simulink model "LoFT_Example3"  (R2024b)
settings: Solver=ode4  StartTime=0.0  StopTime=300  FixedStep=simu.dt  RelTol=1e-3
undefined symbols (not defined in the file): body, circtime, Communication, D1, Delta, irkb, line, LoFT, p0, Pn, s, simu, trip_time, Turbwind, waves, wind
libraries: simulink x350, spsThreePhaseVIMeasurementLib x41, spsThreePhasePISectionLineLib x34, spsThreePhaseParallelRLCLoadLib x21, spsThreePhaseTransformerTwoWindingsLib x14, spsLoadFlowBusLib x10, spsThreePhaseDynamicLoadLib x9, spsSynchronousMachinepuStandardLib x7, spsExcitationSystemLib x7, spsSteamTurbineandGovernorLib x7, spsGenericPowerSystemStabilizerLib x7, spsMultiBandPowerSystemStabilizerLib x7
(part 48 of 49)

== system LoFT_Example3/Onshore grid/Onshore Grid/Subsystem/SG9/Regulators9/Turbine  & Excitation Regulators Mac2/Stabilisateur ==
  Pm : Inport
  Pe : Inport  Port=2
  dw : Inport  Port=3
  Generic Power System Stabilizer : spsGenericPowerSystemStabilizerLib/Generic Power System Stabilizer  Tsensor=15e-3  K=2.5  Twashout=1  Tleadlag1="[0.06  1]"  Tleadlag2="[0  0]"  VSlimits=[-0.15 0.15]  Vinit=0  Plot_On=off  MagdB_On=on  FreqRange=logspace(-2,2,500)
  Ground1 : Ground
  Multi-Band Power System Stabilizer : spsMultiBandPowerSystemStabilizerLib/Multi-Band Power System Stabilizer  OperationMode=Simplified settings  Kg=0.7  GL=[0.2 10]  GI=[0.9 30]  GH=[12.0 115]  GLd=[66 66 9.4]  TcLF=[1.667 2 0 0 0 0 2 2.4 0 0 0 0 1 1]  GId=[66 66 47.6]  TcIF=[1 1 0.25 0.3 0 0 1 1 0.3 0.36 0 0 0 0]  GHd=[66 66 233]  TcHF="[0.01 0.012 0 0 0 0  0.012 0.0144 0 0 0 0 1 1]"  LIM=[.075 .15 .15 .15]  Plot_On=off  MagdB_On=on  FreqRange=logspace(-2,2,500)
  Multiport Switch : MultiPortSwitch
  Sum2 : Sum  Inputs=+-  InputSameDT=on  SaturateOnIntegerOverflow=on  OutDataTypeStr=Inherit: Same as first input
  Stab : Outport  InitialOutput=0  VectorParamsAs1DForOutWhenUnconnected=off
  wires:
  Multi-Band Power System Stabilizer/1 -> Multiport Switch/4
  dw/1 -> Multi-Band Power System Stabilizer/1
  [PSS_select] -> Multiport Switch/1
  Ground1/1 -> Multiport Switch/2
  Pe/1 -> Sum2/2
  Pm/1 -> Sum2/1
  Sum2/1 -> Generic Power System Stabilizer/1
  Generic Power System Stabilizer/1 -> Multiport Switch/3
  Multiport Switch/1 -> Stab/1

== matlab function LoFT_Example3/FOWT System/Subsystem7/FOWT1/Hydrodynamics/radiation force/MATLAB Function ==
  data: velocity input; radiationdamping output; irkb input; circtime input
function radiationdamping  = fcn(velocity,irkb,circtime)

radiationdamping  = ConvolutionIntegral_interp(velocity,irkb,circtime);
end

== matlab function LoFT_Example3/FOWT System/Subsystem7/FOWT10/Hydrodynamics/excitation force/WECSim Linear wave excitiation ==
  data: A input; Fext output; w input; fExtRE input; fExtIM input; phaseRand input; dw input; time input; WaveDir input; spread input; fExtMD input
function Fext = irregExcF(A,w,fExtRE,fExtIM,phaseRand,dw,time,WaveDir,spread,fExtMD)

Fext = irregExcF(A,w,fExtRE,fExtIM,phaseRand,dw,time,WaveDir,spread,fExtMD);

end

== matlab function LoFT_Example3/FOWT System/Subsystem7/FOWT10/Hydrodynamics/radiation force/MATLAB Function ==
  data: velocity input; radiationdamping output; irkb input; circtime input
function radiationdamping  = fcn(velocity,irkb,circtime)

radiationdamping  = ConvolutionIntegral_interp(velocity,irkb,circtime);
end

== matlab function LoFT_Example3/FOWT System/Subsystem7/FOWT2/Hydrodynamics/excitation force/WECSim Linear wave excitiation ==
  data: A input; Fext output; w input; fExtRE input; fExtIM input; phaseRand input; dw input; time input; WaveDir input; spread input; fExtMD input
function Fext = irregExcF(A,w,fExtRE,fExtIM,phaseRand,dw,time,WaveDir,spread,fExtMD)

Fext = irregExcF(A,w,fExtRE,fExtIM,phaseRand,dw,time,WaveDir,spread,fExtMD);

end

== matlab function LoFT_Example3/FOWT System/Subsystem7/FOWT2/Hydrodynamics/radiation force/MATLAB Function ==
  data: velocity input; radiationdamping output; irkb input; circtime input
function radiationdamping  = fcn(velocity,irkb,circtime)

radiationdamping  = ConvolutionIntegral_interp(velocity,irkb,circtime);
end

== matlab function LoFT_Example3/FOWT System/Subsystem7/FOWT3/Hydrodynamics/excitation force/WECSim Linear wave excitiation ==
  data: A input; Fext output; w input; fExtRE input; fExtIM input; phaseRand input; dw input; time input; WaveDir input; spread input; fExtMD input
function Fext = irregExcF(A,w,fExtRE,fExtIM,phaseRand,dw,time,WaveDir,spread,fExtMD)

Fext = irregExcF(A,w,fExtRE,fExtIM,phaseRand,dw,time,WaveDir,spread,fExtMD);

end

== matlab function LoFT_Example3/FOWT System/Subsystem1/FOWT5/Hydrodynamics/radiation force/MATLAB Function ==
  data: velocity input; radiationdamping output; irkb input; circtime input
function radiationdamping  = fcn(velocity,irkb,circtime)

radiationdamping  = ConvolutionIntegral_interp(velocity,irkb,circtime);
end

== matlab function LoFT_Example3/FOWT System/Subsystem7/FOWT3/Hydrodynamics/radiation force/MATLAB Function ==
  data: velocity input; radiationdamping output; irkb input; circtime input
function radiationdamping  = fcn(velocity,irkb,circtime)

radiationdamping  = ConvolutionIntegral_interp(velocity,irkb,circtime);
end

== matlab function LoFT_Example3/FOWT System/Subsystem7/FOWT4/Hydrodynamics/excitation force/WECSim Linear wave excitiation ==
  data: A input; Fext output; w input; fExtRE input; fExtIM input; phaseRand input; dw input; time input; WaveDir input; spread input; fExtMD input
function Fext = irregExcF(A,w,fExtRE,fExtIM,phaseRand,dw,time,WaveDir,spread,fExtMD)

Fext = irregExcF(A,w,fExtRE,fExtIM,phaseRand,dw,time,WaveDir,spread,fExtMD);

end

== matlab function LoFT_Example3/FOWT System/Subsystem7/FOWT4/Hydrodynamics/radiation force/MATLAB Function ==
  data: velocity input; radiationdamping output; irkb input; circtime input
function radiationdamping  = fcn(velocity,irkb,circtime)

radiationdamping  = ConvolutionIntegral_interp(velocity,irkb,circtime);
end

== matlab function LoFT_Example3/FOWT System/Subsystem7/FOWT5/Hydrodynamics/excitation force/WECSim Linear wave excitiation ==
  data: A input; Fext output; w input; fExtRE input; fExtIM input; phaseRand input; dw input; time input; WaveDir input; spread input; fExtMD input
function Fext = irregExcF(A,w,fExtRE,fExtIM,phaseRand,dw,time,WaveDir,spread,fExtMD)

Fext = irregExcF(A,w,fExtRE,fExtIM,phaseRand,dw,time,WaveDir,spread,fExtMD);

end

== matlab function LoFT_Example3/FOWT System/Subsystem7/FOWT5/Hydrodynamics/radiation force/MATLAB Function ==
  data: velocity input; radiationdamping output; irkb input; circtime input
function radiationdamping  = fcn(velocity,irkb,circtime)

radiationdamping  = ConvolutionIntegral_interp(velocity,irkb,circtime);
end

== matlab function LoFT_Example3/FOWT System/Subsystem7/FOWT6/Hydrodynamics/excitation force/WECSim Linear wave excitiation ==
  data: A input; Fext output; w input; fExtRE input; fExtIM input; phaseRand input; dw input; time input; WaveDir input; spread input; fExtMD input
function Fext = irregExcF(A,w,fExtRE,fExtIM,phaseRand,dw,time,WaveDir,spread,fExtMD)

Fext = irregExcF(A,w,fExtRE,fExtIM,phaseRand,dw,time,WaveDir,spread,fExtMD);

end

== matlab function LoFT_Example3/FOWT System/Subsystem7/FOWT6/Hydrodynamics/radiation force/MATLAB Function ==
  data: velocity input; radiationdamping output; irkb input; circtime input
function radiationdamping  = fcn(velocity,irkb,circtime)

radiationdamping  = ConvolutionIntegral_interp(velocity,irkb,circtime);
end

== matlab function LoFT_Example3/FOWT System/Subsystem1/FOWT6/Hydrodynamics/excitation force/WECSim Linear wave excitiation ==
  data: A input; Fext output; w input; fExtRE input; fExtIM input; phaseRand input; dw input; time input; WaveDir input; spread input; fExtMD input
function Fext = irregExcF(A,w,fExtRE,fExtIM,phaseRand,dw,time,WaveDir,spread,fExtMD)

Fext = irregExcF(A,w,fExtRE,fExtIM,phaseRand,dw,time,WaveDir,spread,fExtMD);

end

== matlab function LoFT_Example3/FOWT System/Subsystem7/FOWT7/Hydrodynamics/excitation force/WECSim Linear wave excitiation ==
  data: A input; Fext output; w input; fExtRE input; fExtIM input; phaseRand input; dw input; time input; WaveDir input; spread input; fExtMD input
function Fext = irregExcF(A,w,fExtRE,fExtIM,phaseRand,dw,time,WaveDir,spread,fExtMD)

Fext = irregExcF(A,w,fExtRE,fExtIM,phaseRand,dw,time,WaveDir,spread,fExtMD);

end

== matlab function LoFT_Example3/FOWT System/Subsystem7/FOWT7/Hydrodynamics/radiation force/MATLAB Function ==
  data: velocity input; radiationdamping output; irkb input; circtime input
function radiationdamping  = fcn(velocity,irkb,circtime)

radiationdamping  = ConvolutionIntegral_interp(velocity,irkb,circtime);
end

== matlab function LoFT_Example3/FOWT System/Subsystem7/FOWT8/Hydrodynamics/excitation force/WECSim Linear wave excitiation ==
  data: A input; Fext output; w input; fExtRE input; fExtIM input; phaseRand input; dw input; time input; WaveDir input; spread input; fExtMD input
function Fext = irregExcF(A,w,fExtRE,fExtIM,phaseRand,dw,time,WaveDir,spread,fExtMD)

Fext = irregExcF(A,w,fExtRE,fExtIM,phaseRand,dw,time,WaveDir,spread,fExtMD);

end

== matlab function LoFT_Example3/FOWT System/Subsystem7/FOWT8/Hydrodynamics/radiation force/MATLAB Function ==
  data: velocity input; radiationdamping output; irkb input; circtime input
function radiationdamping  = fcn(velocity,irkb,circtime)

radiationdamping  = ConvolutionIntegral_interp(velocity,irkb,circtime);
end

== matlab function LoFT_Example3/FOWT System/Subsystem7/FOWT9/Hydrodynamics/excitation force/WECSim Linear wave excitiation ==
  data: A input; Fext output; w input; fExtRE input; fExtIM input; phaseRand input; dw input; time input; WaveDir input; spread input; fExtMD input
function Fext = irregExcF(A,w,fExtRE,fExtIM,phaseRand,dw,time,WaveDir,spread,fExtMD)

Fext = irregExcF(A,w,fExtRE,fExtIM,phaseRand,dw,time,WaveDir,spread,fExtMD);

end

== matlab function LoFT_Example3/FOWT System/Subsystem7/FOWT9/Hydrodynamics/radiation force/MATLAB Function ==
  data: velocity input; radiationdamping output; irkb input; circtime input
function radiationdamping  = fcn(velocity,irkb,circtime)

radiationdamping  = ConvolutionIntegral_interp(velocity,irkb,circtime);
end

== matlab function LoFT_Example3/FOWT System/Subsystem11/FOWT1/Hydrodynamics/excitation force/WECSim Linear wave excitiation ==
  data: A input; Fext output; w input; fExtRE input; fExtIM input; phaseRand input; dw input; time input; WaveDir input; spread input; fExtMD input
function Fext = irregExcF(A,w,fExtRE,fExtIM,phaseRand,dw,time,WaveDir,spread,fExtMD)

Fext = irregExcF(A,w,fExtRE,fExtIM,phaseRand,dw,time,WaveDir,spread,fExtMD);

end

== matlab function LoFT_Example3/FOWT System/Subsystem11/FOWT1/Hydrodynamics/radiation force/MATLAB Function ==
  data: velocity input; radiationdamping output; irkb input; circtime input
function radiationdamping  = fcn(velocity,irkb,circtime)

radiationdamping  = ConvolutionIntegral_interp(velocity,irkb,circtime);
end

== matlab function LoFT_Example3/FOWT System/Subsystem11/FOWT10/Hydrodynamics/excitation force/WECSim Linear wave excitiation ==
  data: A input; Fext output; w input; fExtRE input; fExtIM input; phaseRand input; dw input; time input; WaveDir input; spread input; fExtMD input
function Fext = irregExcF(A,w,fExtRE,fExtIM,phaseRand,dw,time,WaveDir,spread,fExtMD)

Fext = irregExcF(A,w,fExtRE,fExtIM,phaseRand,dw,time,WaveDir,spread,fExtMD);

end

== matlab function LoFT_Example3/FOWT System/Subsystem11/FOWT10/Hydrodynamics/radiation force/MATLAB Function ==
  data: velocity input; radiationdamping output; irkb input; circtime input
function radiationdamping  = fcn(velocity,irkb,circtime)

radiationdamping  = ConvolutionIntegral_interp(velocity,irkb,circtime);
end

== matlab function LoFT_Example3/FOWT System/Subsystem11/FOWT2/Hydrodynamics/excitation force/WECSim Linear wave excitiation ==
  data: A input; Fext output; w input; fExtRE input; fExtIM input; phaseRand input; dw input; time input; WaveDir input; spread input; fExtMD input
function Fext = irregExcF(A,w,fExtRE,fExtIM,phaseRand,dw,time,WaveDir,spread,fExtMD)

Fext = irregExcF(A,w,fExtRE,fExtIM,phaseRand,dw,time,WaveDir,spread,fExtMD);

end

== matlab function LoFT_Example3/FOWT System/Subsystem11/FOWT2/Hydrodynamics/radiation force/MATLAB Function ==
  data: velocity input; radiationdamping output; irkb input; circtime input
function radiationdamping  = fcn(velocity,irkb,circtime)

radiationdamping  = ConvolutionIntegral_interp(velocity,irkb,circtime);
end

== matlab function LoFT_Example3/FOWT System/Subsystem11/FOWT3/Hydrodynamics/excitation force/WECSim Linear wave excitiation ==
  data: A input; Fext output; w input; fExtRE input; fExtIM input; phaseRand input; dw input; time input; WaveDir input; spread input; fExtMD input
function Fext = irregExcF(A,w,fExtRE,fExtIM,phaseRand,dw,time,WaveDir,spread,fExtMD)

Fext = irregExcF(A,w,fExtRE,fExtIM,phaseRand,dw,time,WaveDir,spread,fExtMD);

end

== matlab function LoFT_Example3/FOWT System/Subsystem1/FOWT6/Hydrodynamics/radiation force/MATLAB Function ==
  data: velocity input; radiationdamping output; irkb input; circtime input
function radiationdamping  = fcn(velocity,irkb,circtime)

radiationdamping  = ConvolutionIntegral_interp(velocity,irkb,circtime);
end

== matlab function LoFT_Example3/FOWT System/Subsystem11/FOWT3/Hydrodynamics/radiation force/MATLAB Function ==
  data: velocity input; radiationdamping output; irkb input; circtime input
function radiationdamping  = fcn(velocity,irkb,circtime)

radiationdamping  = ConvolutionIntegral_interp(velocity,irkb,circtime);
end

== matlab function LoFT_Example3/FOWT System/Subsystem11/FOWT4/Hydrodynamics/excitation force/WECSim Linear wave excitiation ==
  data: A input; Fext output; w input; fExtRE input; fExtIM input; phaseRand input; dw input; time input; WaveDir input; spread input; fExtMD input
function Fext = irregExcF(A,w,fExtRE,fExtIM,phaseRand,dw,time,WaveDir,spread,fExtMD)

Fext = irregExcF(A,w,fExtRE,fExtIM,phaseRand,dw,time,WaveDir,spread,fExtMD);

end

== matlab function LoFT_Example3/FOWT System/Subsystem11/FOWT4/Hydrodynamics/radiation force/MATLAB Function ==
  data: velocity input; radiationdamping output; irkb input; circtime input
function radiationdamping  = fcn(velocity,irkb,circtime)

radiationdamping  = ConvolutionIntegral_interp(velocity,irkb,circtime);
end

== matlab function LoFT_Example3/FOWT System/Subsystem11/FOWT5/Hydrodynamics/excitation force/WECSim Linear wave excitiation ==
  data: A input; Fext output; w input; fExtRE input; fExtIM input; phaseRand input; dw input; time input; WaveDir input; spread input; fExtMD input
function Fext = irregExcF(A,w,fExtRE,fExtIM,phaseRand,dw,time,WaveDir,spread,fExtMD)

Fext = irregExcF(A,w,fExtRE,fExtIM,phaseRand,dw,time,WaveDir,spread,fExtMD);

end

== matlab function LoFT_Example3/FOWT System/Subsystem11/FOWT5/Hydrodynamics/radiation force/MATLAB Function ==
  data: velocity input; radiationdamping output; irkb input; circtime input
function radiationdamping  = fcn(velocity,irkb,circtime)

radiationdamping  = ConvolutionIntegral_interp(velocity,irkb,circtime);
end

== matlab function LoFT_Example3/FOWT System/Subsystem11/FOWT6/Hydrodynamics/excitation force/WECSim Linear wave excitiation ==
  data: A input; Fext output; w input; fExtRE input; fExtIM input; phaseRand input; dw input; time input; WaveDir input; spread input; fExtMD input
function Fext = irregExcF(A,w,fExtRE,fExtIM,phaseRand,dw,time,WaveDir,spread,fExtMD)

Fext = irregExcF(A,w,fExtRE,fExtIM,phaseRand,dw,time,WaveDir,spread,fExtMD);

end

== matlab function LoFT_Example3/FOWT System/Subsystem11/FOWT6/Hydrodynamics/radiation force/MATLAB Function ==
  data: velocity input; radiationdamping output; irkb input; circtime input
function radiationdamping  = fcn(velocity,irkb,circtime)

radiationdamping  = ConvolutionIntegral_interp(velocity,irkb,circtime);
end

== matlab function LoFT_Example3/FOWT System/Subsystem1/FOWT7/Hydrodynamics/excitation force/WECSim Linear wave excitiation ==
  data: A input; Fext output; w input; fExtRE input; fExtIM input; phaseRand input; dw input; time input; WaveDir input; spread input; fExtMD input
function Fext = irregExcF(A,w,fExtRE,fExtIM,phaseRand,dw,time,WaveDir,spread,fExtMD)

Fext = irregExcF(A,w,fExtRE,fExtIM,phaseRand,dw,time,WaveDir,spread,fExtMD);

end

== matlab function LoFT_Example3/FOWT System/Subsystem11/FOWT7/Hydrodynamics/excitation force/WECSim Linear wave excitiation ==
  data: A input; Fext output; w input; fExtRE input; fExtIM input; phaseRand input; dw input; time input; WaveDir input; spread input; fExtMD input
function Fext = irregExcF(A,w,fExtRE,fExtIM,phaseRand,dw,time,WaveDir,spread,fExtMD)

Fext = irregExcF(A,w,fExtRE,fExtIM,phaseRand,dw,time,WaveDir,spread,fExtMD);

end

== matlab function LoFT_Example3/FOWT System/Subsystem11/FOWT7/Hydrodynamics/radiation force/MATLAB Function ==
  data: velocity input; radiationdamping output; irkb input; circtime input
function radiationdamping  = fcn(velocity,irkb,circtime)

radiationdamping  = ConvolutionIntegral_interp(velocity,irkb,circtime);
end

== matlab function LoFT_Example3/FOWT System/Subsystem11/FOWT8/Hydrodynamics/excitation force/WECSim Linear wave excitiation ==
  data: A input; Fext output; w input; fExtRE input; fExtIM input; phaseRand input; dw input; time input; WaveDir input; spread input; fExtMD input
function Fext = irregExcF(A,w,fExtRE,fExtIM,phaseRand,dw,time,WaveDir,spread,fExtMD)

Fext = irregExcF(A,w,fExtRE,fExtIM,phaseRand,dw,time,WaveDir,spread,fExtMD);

end

== matlab function LoFT_Example3/FOWT System/Subsystem11/FOWT8/Hydrodynamics/radiation force/MATLAB Function ==
  data: velocity input; radiationdamping output; irkb input; circtime input
function radiationdamping  = fcn(velocity,irkb,circtime)

radiationdamping  = ConvolutionIntegral_interp(velocity,irkb,circtime);
end

== matlab function LoFT_Example3/FOWT System/Subsystem11/FOWT9/Hydrodynamics/excitation force/WECSim Linear wave excitiation ==
  data: A input; Fext output; w input; fExtRE input; fExtIM input; phaseRand input; dw input; time input; WaveDir input; spread input; fExtMD input
function Fext = irregExcF(A,w,fExtRE,fExtIM,phaseRand,dw,time,WaveDir,spread,fExtMD)

Fext = irregExcF(A,w,fExtRE,fExtIM,phaseRand,dw,time,WaveDir,spread,fExtMD);

end

== matlab function LoFT_Example3/FOWT System/Subsystem11/FOWT9/Hydrodynamics/radiation force/MATLAB Function ==
  data: velocity input; radiationdamping output; irkb input; circtime input
function radiationdamping  = fcn(velocity,irkb,circtime)

radiationdamping  = ConvolutionIntegral_interp(velocity,irkb,circtime);
end

== matlab function LoFT_Example3/FOWT System/Subsystem13/FOWT1/Hydrodynamics/excitation force/WECSim Linear wave excitiation ==
  data: A input; Fext output; w input; fExtRE input; fExtIM input; phaseRand input; dw input; time input; WaveDir input; spread input; fExtMD input
function Fext = irregExcF(A,w,fExtRE,fExtIM,phaseRand,dw,time,WaveDir,spread,fExtMD)

Fext = irregExcF(A,w,fExtRE,fExtIM,phaseRand,dw,time,WaveDir,spread,fExtMD);

end

== matlab function LoFT_Example3/FOWT System/Subsystem13/FOWT1/Hydrodynamics/radiation force/MATLAB Function ==
  data: velocity input; radiationdamping output; irkb input; circtime input
function radiationdamping  = fcn(velocity,irkb,circtime)

radiationdamping  = ConvolutionIntegral_interp(velocity,irkb,circtime);
end

== matlab function LoFT_Example3/FOWT System/Subsystem13/FOWT10/Hydrodynamics/excitation force/WECSim Linear wave excitiation ==
  data: A input; Fext output; w input; fExtRE input; fExtIM input; phaseRand input; dw input; time input; WaveDir input; spread input; fExtMD input
function Fext = irregExcF(A,w,fExtRE,fExtIM,phaseRand,dw,time,WaveDir,spread,fExtMD)

Fext = irregExcF(A,w,fExtRE,fExtIM,phaseRand,dw,time,WaveDir,spread,fExtMD);

end

== matlab function LoFT_Example3/FOWT System/Subsystem13/FOWT10/Hydrodynamics/radiation force/MATLAB Function ==
  data: velocity input; radiationdamping output; irkb input; circtime input
function radiationdamping  = fcn(velocity,irkb,circtime)

radiationdamping  = ConvolutionIntegral_interp(velocity,irkb,circtime);
end

== matlab function LoFT_Example3/FOWT System/Subsystem13/FOWT2/Hydrodynamics/excitation force/WECSim Linear wave excitiation ==
  data: A input; Fext output; w input; fExtRE input; fExtIM input; phaseRand input; dw input; time input; WaveDir input; spread input; fExtMD input
function Fext = irregExcF(A,w,fExtRE,fExtIM,phaseRand,dw,time,WaveDir,spread,fExtMD)

Fext = irregExcF(A,w,fExtRE,fExtIM,phaseRand,dw,time,WaveDir,spread,fExtMD);

end

== matlab function LoFT_Example3/FOWT System/Subsystem13/FOWT2/Hydrodynamics/radiation force/MATLAB Function ==
  data: velocity input; radiationdamping output; irkb input; circtime input
function radiationdamping  = fcn(velocity,irkb,circtime)

radiationdamping  = ConvolutionIntegral_interp(velocity,irkb,circtime);
end

== matlab function LoFT_Example3/FOWT System/Subsystem13/FOWT3/Hydrodynamics/excitation force/WECSim Linear wave excitiation ==
  data: A input; Fext output; w input; fExtRE input; fExtIM input; phaseRand input; dw input; time input; WaveDir input; spread input; fExtMD input
function Fext = irregExcF(A,w,fExtRE,fExtIM,phaseRand,dw,time,WaveDir,spread,fExtMD)

Fext = irregExcF(A,w,fExtRE,fExtIM,phaseRand,dw,time,WaveDir,spread,fExtMD);

end

== matlab function LoFT_Example3/FOWT System/Subsystem1/FOWT7/Hydrodynamics/radiation force/MATLAB Function ==
  data: velocity input; radiationdamping output; irkb input; circtime input
function radiationdamping  = fcn(velocity,irkb,circtime)

radiationdamping  = ConvolutionIntegral_interp(velocity,irkb,circtime);
end

== matlab function LoFT_Example3/FOWT System/Subsystem13/FOWT3/Hydrodynamics/radiation force/MATLAB Function ==
  data: velocity input; radiationdamping output; irkb input; circtime input
function radiationdamping  = fcn(velocity,irkb,circtime)

radiationdamping  = ConvolutionIntegral_interp(velocity,irkb,circtime);
end

== matlab function LoFT_Example3/FOWT System/Subsystem13/FOWT4/Hydrodynamics/excitation force/WECSim Linear wave excitiation ==
  data: A input; Fext output; w input; fExtRE input; fExtIM input; phaseRand input; dw input; time input; WaveDir input; spread input; fExtMD input
function Fext = irregExcF(A,w,fExtRE,fExtIM,phaseRand,dw,time,WaveDir,spread,fExtMD)

Fext = irregExcF(A,w,fExtRE,fExtIM,phaseRand,dw,time,WaveDir,spread,fExtMD);

end

== matlab function LoFT_Example3/FOWT System/Subsystem1/FOWT2/Hydrodynamics/excitation force/WECSim Linear wave excitiation ==
  data: A input; Fext output; w input; fExtRE input; fExtIM input; phaseRand input; dw input; time input; WaveDir input; spread input; fExtMD input
function Fext = irregExcF(A,w,fExtRE,fExtIM,phaseRand,dw,time,WaveDir,spread,fExtMD)

Fext = irregExcF(A,w,fExtRE,fExtIM,phaseRand,dw,time,WaveDir,spread,fExtMD);

end

== matlab function LoFT_Example3/FOWT System/Subsystem13/FOWT4/Hydrodynamics/radiation force/MATLAB Function ==
  data: velocity input; radiationdamping output; irkb input; circtime input
function radiationdamping  = fcn(velocity,irkb,circtime)

radiationdamping  = ConvolutionIntegral_interp(velocity,irkb,circtime);
end

== matlab function LoFT_Example3/FOWT System/Subsystem13/FOWT5/Hydrodynamics/excitation force/WECSim Linear wave excitiation ==
  data: A input; Fext output; w input; fExtRE input; fExtIM input; phaseRand input; dw input; time input; WaveDir input; spread input; fExtMD input
function Fext = irregExcF(A,w,fExtRE,fExtIM,phaseRand,dw,time,WaveDir,spread,fExtMD)

Fext = irregExcF(A,w,fExtRE,fExtIM,phaseRand,dw,time,WaveDir,spread,fExtMD);

end

== matlab function LoFT_Example3/FOWT System/Subsystem13/FOWT5/Hydrodynamics/radiation force/MATLAB Function ==
  data: velocity input; radiationdamping output; irkb input; circtime input
function radiationdamping  = fcn(velocity,irkb,circtime)

radiationdamping  = ConvolutionIntegral_interp(velocity,irkb,circtime);
end

== matlab function LoFT_Example3/FOWT System/Subsystem13/FOWT6/Hydrodynamics/excitation force/WECSim Linear wave excitiation ==
  data: A input; Fext output; w input; fExtRE input; fExtIM input; phaseRand input; dw input; time input; WaveDir input; spread input; fExtMD input
function Fext = irregExcF(A,w,fExtRE,fExtIM,phaseRand,dw,time,WaveDir,spread,fExtMD)

Fext = irregExcF(A,w,fExtRE,fExtIM,phaseRand,dw,time,WaveDir,spread,fExtMD);

end

== matlab function LoFT_Example3/FOWT System/Subsystem13/FOWT6/Hydrodynamics/radiation force/MATLAB Function ==
  data: velocity input; radiationdamping output; irkb input; circtime input
function radiationdamping  = fcn(velocity,irkb,circtime)

radiationdamping  = ConvolutionIntegral_interp(velocity,irkb,circtime);
end

== matlab function LoFT_Example3/FOWT System/Subsystem1/FOWT8/Hydrodynamics/excitation force/WECSim Linear wave excitiation ==
  data: A input; Fext output; w input; fExtRE input; fExtIM input; phaseRand input; dw input; time input; WaveDir input; spread input; fExtMD input
function Fext = irregExcF(A,w,fExtRE,fExtIM,phaseRand,dw,time,WaveDir,spread,fExtMD)

Fext = irregExcF(A,w,fExtRE,fExtIM,phaseRand,dw,time,WaveDir,spread,fExtMD);

end

== matlab function LoFT_Example3/FOWT System/Subsystem13/FOWT7/Hydrodynamics/excitation force/WECSim Linear wave excitiation ==
  data: A input; Fext output; w input; fExtRE input; fExtIM input; phaseRand input; dw input; time input; WaveDir input; spread input; fExtMD input
function Fext = irregExcF(A,w,fExtRE,fExtIM,phaseRand,dw,time,WaveDir,spread,fExtMD)

Fext = irregExcF(A,w,fExtRE,fExtIM,phaseRand,dw,time,WaveDir,spread,fExtMD);

end

== matlab function LoFT_Example3/FOWT System/Subsystem13/FOWT7/Hydrodynamics/radiation force/MATLAB Function ==
  data: velocity input; radiationdamping output; irkb input; circtime input
function radiationdamping  = fcn(velocity,irkb,circtime)

radiationdamping  = ConvolutionIntegral_interp(velocity,irkb,circtime);
end

== matlab function LoFT_Example3/FOWT System/Subsystem13/FOWT8/Hydrodynamics/excitation force/WECSim Linear wave excitiation ==
  data: A input; Fext output; w input; fExtRE input; fExtIM input; phaseRand input; dw input; time input; WaveDir input; spread input; fExtMD input
function Fext = irregExcF(A,w,fExtRE,fExtIM,phaseRand,dw,time,WaveDir,spread,fExtMD)

Fext = irregExcF(A,w,fExtRE,fExtIM,phaseRand,dw,time,WaveDir,spread,fExtMD);

end

== matlab function LoFT_Example3/FOWT System/Subsystem13/FOWT8/Hydrodynamics/radiation force/MATLAB Function ==
  data: velocity input; radiationdamping output; irkb input; circtime input
function radiationdamping  = fcn(velocity,irkb,circtime)

radiationdamping  = ConvolutionIntegral_interp(velocity,irkb,circtime);
end

== matlab function LoFT_Example3/FOWT System/Subsystem13/FOWT9/Hydrodynamics/excitation force/WECSim Linear wave excitiation ==
  data: A input; Fext output; w input; fExtRE input; fExtIM input; phaseRand input; dw input; time input; WaveDir input; spread input; fExtMD input
function Fext = irregExcF(A,w,fExtRE,fExtIM,phaseRand,dw,time,WaveDir,spread,fExtMD)

Fext = irregExcF(A,w,fExtRE,fExtIM,phaseRand,dw,time,WaveDir,spread,fExtMD);

end

== matlab function LoFT_Example3/FOWT System/Subsystem13/FOWT9/Hydrodynamics/radiation force/MATLAB Function ==
  data: velocity input; radiationdamping output; irkb input; circtime input
function radiationdamping  = fcn(velocity,irkb,circtime)

radiationdamping  = ConvolutionIntegral_interp(velocity,irkb,circtime);
end

== matlab function LoFT_Example3/FOWT System/Subsystem1/FOWT1/Hydrodynamics/excitation force/WECSim Linear wave excitiation ==
  data: A input; Fext output; w input; fExtRE input; fExtIM input; phaseRand input; dw input; time input; WaveDir input; spread input; fExtMD input
function Fext = irregExcF(A,w,fExtRE,fExtIM,phaseRand,dw,time,WaveDir,spread,fExtMD)

Fext = irregExcF(A,w,fExtRE,fExtIM,phaseRand,dw,time,WaveDir,spread,fExtMD);

end

== matlab function LoFT_Example3/FOWT System/Subsystem1/FOWT1/Hydrodynamics/radiation force/MATLAB Function ==
  data: velocity input; radiationdamping output; irkb input; circtime input
function radiationdamping  = fcn(velocity,irkb,circtime)

radiationdamping  = ConvolutionIntegral_interp(velocity,irkb,circtime);
end

== matlab function LoFT_Example3/FOWT System/Subsystem1/FOWT8/Hydrodynamics/radiation force/MATLAB Function ==
  data: velocity input; radiationdamping output; irkb input; circtime input
function radiationdamping  = fcn(velocity,irkb,circtime)

radiationdamping  = ConvolutionIntegral_interp(velocity,irkb,circtime);
end

== matlab function LoFT_Example3/FOWT System/Subsystem1/FOWT9/Hydrodynamics/excitation force/WECSim Linear wave excitiation ==
  data: A input; Fext output; w input; fExtRE input; fExtIM input; phaseRand input; dw input; time input; WaveDir input; spread input; fExtMD input
function Fext = irregExcF(A,w,fExtRE,fExtIM,phaseRand,dw,time,WaveDir,spread,fExtMD)

Fext = irregExcF(A,w,fExtRE,fExtIM,phaseRand,dw,time,WaveDir,spread,fExtMD);

end

== matlab function LoFT_Example3/FOWT System/Subsystem1/FOWT9/Hydrodynamics/radiation force/MATLAB Function ==
  data: velocity input; radiationdamping output; irkb input; circtime input
function radiationdamping  = fcn(velocity,irkb,circtime)

radiationdamping  = ConvolutionIntegral_interp(velocity,irkb,circtime);
end

== matlab function LoFT_Example3/FOWT System/Subsystem1/FOWT10/Hydrodynamics/excitation force/WECSim Linear wave excitiation ==
  data: A input; Fext output; w input; fExtRE input; fExtIM input; phaseRand input; dw input; time input; WaveDir input; spread input; fExtMD input
function Fext = irregExcF(A,w,fExtRE,fExtIM,phaseRand,dw,time,WaveDir,spread,fExtMD)

Fext = irregExcF(A,w,fExtRE,fExtIM,phaseRand,dw,time,WaveDir,spread,fExtMD);

end

== matlab function LoFT_Example3/FOWT System/Subsystem1/FOWT10/Hydrodynamics/radiation force/MATLAB Function ==
  data: velocity input; radiationdamping output; irkb input; circtime input
function radiationdamping  = fcn(velocity,irkb,circtime)

radiationdamping  = ConvolutionIntegral_interp(velocity,irkb,circtime);
end

== matlab function LoFT_Example3/FOWT System/Subsystem2/FOWT1/Hydrodynamics/excitation force/WECSim Linear wave excitiation ==
  data: A input; Fext output; w input; fExtRE input; fExtIM input; phaseRand input; dw input; time input; WaveDir input; spread input; fExtMD input
function Fext = irregExcF(A,w,fExtRE,fExtIM,phaseRand,dw,time,WaveDir,spread,fExtMD)

Fext = irregExcF(A,w,fExtRE,fExtIM,phaseRand,dw,time,WaveDir,spread,fExtMD);

end

== matlab function LoFT_Example3/FOWT System/Subsystem2/FOWT1/Hydrodynamics/radiation force/MATLAB Function ==
  data: velocity input; radiationdamping output; irkb input; circtime input
function radiationdamping  = fcn(velocity,irkb,circtime)

radiationdamping  = ConvolutionIntegral_interp(velocity,irkb,circtime);
end

== matlab function LoFT_Example3/FOWT System/Subsystem2/FOWT10/Hydrodynamics/excitation force/WECSim Linear wave excitiation ==
  data: A input; Fext output; w input; fExtRE input; fExtIM input; phaseRand input; dw input; time input; WaveDir input; spread input; fExtMD input
function Fext = irregExcF(A,w,fExtRE,fExtIM,phaseRand,dw,time,WaveDir,spread,fExtMD)

Fext = irregExcF(A,w,fExtRE,fExtIM,phaseRand,dw,time,WaveDir,spread,fExtMD);

end

== matlab function LoFT_Example3/FOWT System/Subsystem2/FOWT10/Hydrodynamics/radiation force/MATLAB Function ==
  data: velocity input; radiationdamping output; irkb input; circtime input
function radiationdamping  = fcn(velocity,irkb,circtime)

radiationdamping  = ConvolutionIntegral_interp(velocity,irkb,circtime);
end

== matlab function LoFT_Example3/FOWT System/Subsystem2/FOWT2/Hydrodynamics/excitation force/WECSim Linear wave excitiation ==
  data: A input; Fext output; w input; fExtRE input; fExtIM input; phaseRand input; dw input; time input; WaveDir input; spread input; fExtMD input
function Fext = irregExcF(A,w,fExtRE,fExtIM,phaseRand,dw,time,WaveDir,spread,fExtMD)

Fext = irregExcF(A,w,fExtRE,fExtIM,phaseRand,dw,time,WaveDir,spread,fExtMD);

end

== matlab function LoFT_Example3/FOWT System/Subsystem2/FOWT2/Hydrodynamics/radiation force/MATLAB Function ==
  data: velocity input; radiationdamping output; irkb input; circtime input
function radiationdamping  = fcn(velocity,irkb,circtime)

radiationdamping  = ConvolutionIntegral_interp(velocity,irkb,circtime);
end

== matlab function LoFT_Example3/FOWT System/Subsystem2/FOWT3/Hydrodynamics/excitation force/WECSim Linear wave excitiation ==
  data: A input; Fext output; w input; fExtRE input; fExtIM input; phaseRand input; dw input; time input; WaveDir input; spread input; fExtMD input
function Fext = irregExcF(A,w,fExtRE,fExtIM,phaseRand,dw,time,WaveDir,spread,fExtMD)

Fext = irregExcF(A,w,fExtRE,fExtIM,phaseRand,dw,time,WaveDir,spread,fExtMD);

end

== matlab function LoFT_Example3/FOWT System/Subsystem1/FOWT2/Hydrodynamics/radiation force/MATLAB Function ==
  data: velocity input; radiationdamping output; irkb input; circtime input
function radiationdamping  = fcn(velocity,irkb,circtime)

radiationdamping  = ConvolutionIntegral_interp(velocity,irkb,circtime);
end

== matlab function LoFT_Example3/FOWT System/Subsystem2/FOWT3/Hydrodynamics/radiation force/MATLAB Function ==
  data: velocity input; radiationdamping output; irkb input; circtime input
function radiationdamping  = fcn(velocity,irkb,circtime)

radiationdamping  = ConvolutionIntegral_interp(velocity,irkb,circtime);
end

== matlab function LoFT_Example3/FOWT System/Subsystem2/FOWT4/Hydrodynamics/excitation force/WECSim Linear wave excitiation ==
  data: A input; Fext output; w input; fExtRE input; fExtIM input; phaseRand input; dw input; time input; WaveDir input; spread input; fExtMD input
function Fext = irregExcF(A,w,fExtRE,fExtIM,phaseRand,dw,time,WaveDir,spread,fExtMD)

Fext = irregExcF(A,w,fExtRE,fExtIM,phaseRand,dw,time,WaveDir,spread,fExtMD);

end

== matlab function LoFT_Example3/FOWT System/Subsystem2/FOWT4/Hydrodynamics/radiation force/MATLAB Function ==
  data: velocity input; radiationdamping output; irkb input; circtime input
function radiationdamping  = fcn(velocity,irkb,circtime)

radiationdamping  = ConvolutionIntegral_interp(velocity,irkb,circtime);
end

== matlab function LoFT_Example3/FOWT System/Subsystem2/FOWT5/Hydrodynamics/excitation force/WECSim Linear wave excitiation ==
  data: A input; Fext output; w input; fExtRE input; fExtIM input; phaseRand input; dw input; time input; WaveDir input; spread input; fExtMD input
function Fext = irregExcF(A,w,fExtRE,fExtIM,phaseRand,dw,time,WaveDir,spread,fExtMD)

Fext = irregExcF(A,w,fExtRE,fExtIM,phaseRand,dw,time,WaveDir,spread,fExtMD);

end

== matlab function LoFT_Example3/FOWT System/Subsystem2/FOWT5/Hydrodynamics/radiation force/MATLAB Function ==
  data: velocity input; radiationdamping output; irkb input; circtime input
function radiationdamping  = fcn(velocity,irkb,circtime)

radiationdamping  = ConvolutionIntegral_interp(velocity,irkb,circtime);
end

== matlab function LoFT_Example3/FOWT System/Subsystem2/FOWT6/Hydrodynamics/excitation force/WECSim Linear wave excitiation ==
  data: A input; Fext output; w input; fExtRE input; fExtIM input; phaseRand input; dw input; time input; WaveDir input; spread input; fExtMD input
function Fext = irregExcF(A,w,fExtRE,fExtIM,phaseRand,dw,time,WaveDir,spread,fExtMD)

Fext = irregExcF(A,w,fExtRE,fExtIM,phaseRand,dw,time,WaveDir,spread,fExtMD);

end

== matlab function LoFT_Example3/FOWT System/Subsystem2/FOWT6/Hydrodynamics/radiation force/MATLAB Function ==
  data: velocity input; radiationdamping output; irkb input; circtime input
function radiationdamping  = fcn(velocity,irkb,circtime)

radiationdamping  = ConvolutionIntegral_interp(velocity,irkb,circtime);
end

== matlab function LoFT_Example3/FOWT System/Subsystem1/FOWT3/Hydrodynamics/excitation force/WECSim Linear wave excitiation ==
  data: A input; Fext output; w input; fExtRE input; fExtIM input; phaseRand input; dw input; time input; WaveDir input; spread input; fExtMD input
function Fext = irregExcF(A,w,fExtRE,fExtIM,phaseRand,dw,time,WaveDir,spread,fExtMD)

Fext = irregExcF(A,w,fExtRE,fExtIM,phaseRand,dw,time,WaveDir,spread,fExtMD);

end

== matlab function LoFT_Example3/FOWT System/Subsystem2/FOWT7/Hydrodynamics/excitation force/WECSim Linear wave excitiation ==
  data: A input; Fext output; w input; fExtRE input; fExtIM input; phaseRand input; dw input; time input; WaveDir input; spread input; fExtMD input
function Fext = irregExcF(A,w,fExtRE,fExtIM,phaseRand,dw,time,WaveDir,spread,fExtMD)

Fext = irregExcF(A,w,fExtRE,fExtIM,phaseRand,dw,time,WaveDir,spread,fExtMD);

end

== matlab function LoFT_Example3/FOWT System/Subsystem2/FOWT7/Hydrodynamics/radiation force/MATLAB Function ==
  data: velocity input; radiationdamping output; irkb input; circtime input
function radiationdamping  = fcn(velocity,irkb,circtime)

radiationdamping  = ConvolutionIntegral_interp(velocity,irkb,circtime);
end

== matlab function LoFT_Example3/FOWT System/Subsystem2/FOWT8/Hydrodynamics/excitation force/WECSim Linear wave excitiation ==
  data: A input; Fext output; w input; fExtRE input; fExtIM input; phaseRand input; dw input; time input; WaveDir input; spread input; fExtMD input
function Fext = irregExcF(A,w,fExtRE,fExtIM,phaseRand,dw,time,WaveDir,spread,fExtMD)

Fext = irregExcF(A,w,fExtRE,fExtIM,phaseRand,dw,time,WaveDir,spread,fExtMD);

end

== matlab function LoFT_Example3/FOWT System/Subsystem2/FOWT8/Hydrodynamics/radiation force/MATLAB Function ==
  data: velocity input; radiationdamping output; irkb input; circtime input
function radiationdamping  = fcn(velocity,irkb,circtime)

radiationdamping  = ConvolutionIntegral_interp(velocity,irkb,circtime);
end

== matlab function LoFT_Example3/FOWT System/Subsystem2/FOWT9/Hydrodynamics/excitation force/WECSim Linear wave excitiation ==
  data: A input; Fext output; w input; fExtRE input; fExtIM input; phaseRand input; dw input; time input; WaveDir input; spread input; fExtMD input
function Fext = irregExcF(A,w,fExtRE,fExtIM,phaseRand,dw,time,WaveDir,spread,fExtMD)

Fext = irregExcF(A,w,fExtRE,fExtIM,phaseRand,dw,time,WaveDir,spread,fExtMD);

end

== matlab function LoFT_Example3/FOWT System/Subsystem2/FOWT9/Hydrodynamics/radiation force/MATLAB Function ==
  data: velocity input; radiationdamping output; irkb input; circtime input
function radiationdamping  = fcn(velocity,irkb,circtime)

radiationdamping  = ConvolutionIntegral_interp(velocity,irkb,circtime);
end

== matlab function LoFT_Example3/FOWT System/Subsystem3/FOWT1/Hydrodynamics/excitation force/WECSim Linear wave excitiation ==
  data: A input; Fext output; w input; fExtRE input; fExtIM input; phaseRand input; dw input; time input; WaveDir input; spread input; fExtMD input
function Fext = irregExcF(A,w,fExtRE,fExtIM,phaseRand,dw,time,WaveDir,spread,fExtMD)

Fext = irregExcF(A,w,fExtRE,fExtIM,phaseRand,dw,time,WaveDir,spread,fExtMD);

end

== matlab function LoFT_Example3/FOWT System/Subsystem3/FOWT1/Hydrodynamics/radiation force/MATLAB Function ==
  data: velocity input; radiationdamping output; irkb input; circtime input
function radiationdamping  = fcn(velocity,irkb,circtime)

radiationdamping  = ConvolutionIntegral_interp(velocity,irkb,circtime);
end

== matlab function LoFT_Example3/FOWT System/Subsystem3/FOWT10/Hydrodynamics/excitation force/WECSim Linear wave excitiation ==
  data: A input; Fext output; w input; fExtRE input; fExtIM input; phaseRand input; dw input; time input; WaveDir input; spread input; fExtMD input
function Fext = irregExcF(A,w,fExtRE,fExtIM,phaseRand,dw,time,WaveDir,spread,fExtMD)

Fext = irregExcF(A,w,fExtRE,fExtIM,phaseRand,dw,time,WaveDir,spread,fExtMD);

end

== matlab function LoFT_Example3/FOWT System/Subsystem3/FOWT10/Hydrodynamics/radiation force/MATLAB Function ==
  data: velocity input; radiationdamping output; irkb input; circtime input
function radiationdamping  = fcn(velocity,irkb,circtime)

radiationdamping  = ConvolutionIntegral_interp(velocity,irkb,circtime);
end

== matlab function LoFT_Example3/FOWT System/Subsystem3/FOWT2/Hydrodynamics/excitation force/WECSim Linear wave excitiation ==
  data: A input; Fext output; w input; fExtRE input; fExtIM input; phaseRand input; dw input; time input; WaveDir input; spread input; fExtMD input
function Fext = irregExcF(A,w,fExtRE,fExtIM,phaseRand,dw,time,WaveDir,spread,fExtMD)

Fext = irregExcF(A,w,fExtRE,fExtIM,phaseRand,dw,time,WaveDir,spread,fExtMD);

end

== matlab function LoFT_Example3/FOWT System/Subsystem3/FOWT2/Hydrodynamics/radiation force/MATLAB Function ==
  data: velocity input; radiationdamping output; irkb input; circtime input
function radiationdamping  = fcn(velocity,irkb,circtime)

radiationdamping  = ConvolutionIntegral_interp(velocity,irkb,circtime);
end

== matlab function LoFT_Example3/FOWT System/Subsystem3/FOWT3/Hydrodynamics/excitation force/WECSim Linear wave excitiation ==
  data: A input; Fext output; w input; fExtRE input; fExtIM input; phaseRand input; dw input; time input; WaveDir input; spread input; fExtMD input
function Fext = irregExcF(A,w,fExtRE,fExtIM,phaseRand,dw,time,WaveDir,spread,fExtMD)

Fext = irregExcF(A,w,fExtRE,fExtIM,phaseRand,dw,time,WaveDir,spread,fExtMD);

end

== matlab function LoFT_Example3/FOWT System/Subsystem1/FOWT3/Hydrodynamics/radiation force/MATLAB Function ==
  data: velocity input; radiationdamping output; irkb input; circtime input
function radiationdamping  = fcn(velocity,irkb,circtime)

radiationdamping  = ConvolutionIntegral_interp(velocity,irkb,circtime);
end

== matlab function LoFT_Example3/FOWT System/Subsystem3/FOWT3/Hydrodynamics/radiation force/MATLAB Function ==
  data: velocity input; radiationdamping output; irkb input; circtime input
function radiationdamping  = fcn(velocity,irkb,circtime)

radiationdamping  = ConvolutionIntegral_interp(velocity,irkb,circtime);
end

== matlab function LoFT_Example3/FOWT System/Subsystem3/FOWT4/Hydrodynamics/excitation force/WECSim Linear wave excitiation ==
  data: A input; Fext output; w input; fExtRE input; fExtIM input; phaseRand input; dw input; time input; WaveDir input; spread input; fExtMD input
function Fext = irregExcF(A,w,fExtRE,fExtIM,phaseRand,dw,time,WaveDir,spread,fExtMD)

Fext = irregExcF(A,w,fExtRE,fExtIM,phaseRand,dw,time,WaveDir,spread,fExtMD);

end

== matlab function LoFT_Example3/FOWT System/Subsystem3/FOWT4/Hydrodynamics/radiation force/MATLAB Function ==
  data: velocity input; radiationdamping output; irkb input; circtime input
function radiationdamping  = fcn(velocity,irkb,circtime)

radiationdamping  = ConvolutionIntegral_interp(velocity,irkb,circtime);
end

== matlab function LoFT_Example3/FOWT System/Subsystem3/FOWT5/Hydrodynamics/excitation force/WECSim Linear wave excitiation ==
  data: A input; Fext output; w input; fExtRE input; fExtIM input; phaseRand input; dw input; time input; WaveDir input; spread input; fExtMD input
function Fext = irregExcF(A,w,fExtRE,fExtIM,phaseRand,dw,time,WaveDir,spread,fExtMD)

Fext = irregExcF(A,w,fExtRE,fExtIM,phaseRand,dw,time,WaveDir,spread,fExtMD);

end

== matlab function LoFT_Example3/FOWT System/Subsystem3/FOWT5/Hydrodynamics/radiation force/MATLAB Function ==
  data: velocity input; radiationdamping output; irkb input; circtime input
function radiationdamping  = fcn(velocity,irkb,circtime)

radiationdamping  = ConvolutionIntegral_interp(velocity,irkb,circtime);
end

== matlab function LoFT_Example3/FOWT System/Subsystem3/FOWT6/Hydrodynamics/excitation force/WECSim Linear wave excitiation ==
  data: A input; Fext output; w input; fExtRE input; fExtIM input; phaseRand input; dw input; time input; WaveDir input; spread input; fExtMD input
function Fext = irregExcF(A,w,fExtRE,fExtIM,phaseRand,dw,time,WaveDir,spread,fExtMD)

Fext = irregExcF(A,w,fExtRE,fExtIM,phaseRand,dw,time,WaveDir,spread,fExtMD);

end

== matlab function LoFT_Example3/FOWT System/Subsystem3/FOWT6/Hydrodynamics/radiation force/MATLAB Function ==
  data: velocity input; radiationdamping output; irkb input; circtime input
function radiationdamping  = fcn(velocity,irkb,circtime)

radiationdamping  = ConvolutionIntegral_interp(velocity,irkb,circtime);
end

== matlab function LoFT_Example3/FOWT System/Subsystem1/FOWT4/Hydrodynamics/excitation force/WECSim Linear wave excitiation ==
  data: A input; Fext output; w input; fExtRE input; fExtIM input; phaseRand input; dw input; time input; WaveDir input; spread input; fExtMD input
function Fext = irregExcF(A,w,fExtRE,fExtIM,phaseRand,dw,time,WaveDir,spread,fExtMD)

Fext = irregExcF(A,w,fExtRE,fExtIM,phaseRand,dw,time,WaveDir,spread,fExtMD);

end

== matlab function LoFT_Example3/FOWT System/Subsystem3/FOWT7/Hydrodynamics/excitation force/WECSim Linear wave excitiation ==
  data: A input; Fext output; w input; fExtRE input; fExtIM input; phaseRand input; dw input; time input; WaveDir input; spread input; fExtMD input
function Fext = irregExcF(A,w,fExtRE,fExtIM,phaseRand,dw,time,WaveDir,spread,fExtMD)

Fext = irregExcF(A,w,fExtRE,fExtIM,phaseRand,dw,time,WaveDir,spread,fExtMD);

end

== matlab function LoFT_Example3/FOWT System/Subsystem3/FOWT7/Hydrodynamics/radiation force/MATLAB Function ==
  data: velocity input; radiationdamping output; irkb input; circtime input
function radiationdamping  = fcn(velocity,irkb,circtime)

radiationdamping  = ConvolutionIntegral_interp(velocity,irkb,circtime);
end

== matlab function LoFT_Example3/FOWT System/Subsystem3/FOWT8/Hydrodynamics/excitation force/WECSim Linear wave excitiation ==
  data: A input; Fext output; w input; fExtRE input; fExtIM input; phaseRand input; dw input; time input; WaveDir input; spread input; fExtMD input
function Fext = irregExcF(A,w,fExtRE,fExtIM,phaseRand,dw,time,WaveDir,spread,fExtMD)

Fext = irregExcF(A,w,fExtRE,fExtIM,phaseRand,dw,time,WaveDir,spread,fExtMD);

end

== matlab function LoFT_Example3/FOWT System/Subsystem3/FOWT8/Hydrodynamics/radiation force/MATLAB Function ==
  data: velocity input; radiationdamping output; irkb input; circtime input
function radiationdamping  = fcn(velocity,irkb,circtime)

radiationdamping  = ConvolutionIntegral_interp(velocity,irkb,circtime);
end

== matlab function LoFT_Example3/FOWT System/Subsystem3/FOWT9/Hydrodynamics/excitation force/WECSim Linear wave excitiation ==
  data: A input; Fext output; w input; fExtRE input; fExtIM input; phaseRand input; dw input; time input; WaveDir input; spread input; fExtMD input
function Fext = irregExcF(A,w,fExtRE,fExtIM,phaseRand,dw,time,WaveDir,spread,fExtMD)

Fext = irregExcF(A,w,fExtRE,fExtIM,phaseRand,dw,time,WaveDir,spread,fExtMD);

end

== matlab function LoFT_Example3/FOWT System/Subsystem3/FOWT9/Hydrodynamics/radiation force/MATLAB Function ==
  data: velocity input; radiationdamping output; irkb input; circtime input
function radiationdamping  = fcn(velocity,irkb,circtime)

radiationdamping  = ConvolutionIntegral_interp(velocity,irkb,circtime);
end

== matlab function LoFT_Example3/FOWT System/Subsystem5/FOWT1/Hydrodynamics/excitation force/WECSim Linear wave excitiation ==
  data: A input; Fext output; w input; fExtRE input; fExtIM input; phaseRand input; dw input; time input; WaveDir input; spread input; fExtMD input
function Fext = irregExcF(A,w,fExtRE,fExtIM,phaseRand,dw,time,WaveDir,spread,fExtMD)

Fext = irregExcF(A,w,fExtRE,fExtIM,phaseRand,dw,time,WaveDir,spread,fExtMD);

end

== matlab function LoFT_Example3/FOWT System/Subsystem5/FOWT1/Hydrodynamics/radiation force/MATLAB Function ==
  data: velocity input; radiationdamping output; irkb input; circtime input
function radiationdamping  = fcn(velocity,irkb,circtime)

radiationdamping  = ConvolutionIntegral_interp(velocity,irkb,circtime);
end

== matlab function LoFT_Example3/FOWT System/Subsystem5/FOWT10/Hydrodynamics/excitation force/WECSim Linear wave excitiation ==
  data: A input; Fext output; w input; fExtRE input; fExtIM input; phaseRand input; dw input; time input; WaveDir input; spread input; fExtMD input
function Fext = irregExcF(A,w,fExtRE,fExtIM,phaseRand,dw,time,WaveDir,spread,fExtMD)

Fext = irregExcF(A,w,fExtRE,fExtIM,phaseRand,dw,time,WaveDir,spread,fExtMD);

end

== matlab function LoFT_Example3/FOWT System/Subsystem5/FOWT10/Hydrodynamics/radiation force/MATLAB Function ==
  data: velocity input; radiationdamping output; irkb input; circtime input
function radiationdamping  = fcn(velocity,irkb,circtime)

radiationdamping  = ConvolutionIntegral_interp(velocity,irkb,circtime);
end

== matlab function LoFT_Example3/FOWT System/Subsystem5/FOWT2/Hydrodynamics/excitation force/WECSim Linear wave excitiation ==
  data: A input; Fext output; w input; fExtRE input; fExtIM input; phaseRand input; dw input; time input; WaveDir input; spread input; fExtMD input
function Fext = irregExcF(A,w,fExtRE,fExtIM,phaseRand,dw,time,WaveDir,spread,fExtMD)

Fext = irregExcF(A,w,fExtRE,fExtIM,phaseRand,dw,time,WaveDir,spread,fExtMD);

end

== matlab function LoFT_Example3/FOWT System/Subsystem5/FOWT2/Hydrodynamics/radiation force/MATLAB Function ==
  data: velocity input; radiationdamping output; irkb input; circtime input
function radiationdamping  = fcn(velocity,irkb,circtime)

radiationdamping  = ConvolutionIntegral_interp(velocity,irkb,circtime);
end

== matlab function LoFT_Example3/FOWT System/Subsystem5/FOWT3/Hydrodynamics/excitation force/WECSim Linear wave excitiation ==
  data: A input; Fext output; w input; fExtRE input; fExtIM input; phaseRand input; dw input; time input; WaveDir input; spread input; fExtMD input
function Fext = irregExcF(A,w,fExtRE,fExtIM,phaseRand,dw,time,WaveDir,spread,fExtMD)

Fext = irregExcF(A,w,fExtRE,fExtIM,phaseRand,dw,time,WaveDir,spread,fExtMD);

end
